simulink model "motor_dc"  (R2020b)
settings: Solver=VariableStepAuto  StartTime=0.0  StopTime=0.5  RelTol=1e-3
values from neighbouring files (symbols this model uses):
  b = 1.34e-6    (= 1.34e-06)    [parametres_load.m]
  J = 1.62e-6    (= 1.62e-06)    [parametres_load.m]
  kb = 0.011    [parametres_load.m]
  kt = 0.011    [parametres_load.m]
  La = 0.58e-3    (= 0.00058)    [parametres_load.m]
  Ra = 1.17    [parametres_load.m]
settings Model: Creator=leo7s  LastModifiedBy=leo7s

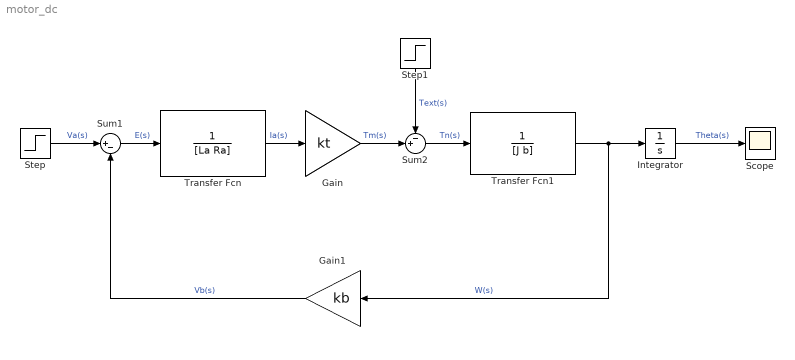
== system motor_dc ==
  Gain : Gain  Gain=kt
  Gain1 : Gain  Gain=kb
  Integrator : Integrator
  Scope : Scope
  Step : Step  Time=0  After=12  SampleTime=0
  Step1 : Step  Time=0  After=0  SampleTime=0
  Sum1 : Sum  Inputs=|+-
  Sum2 : Sum  Inputs=-+|
  Transfer Fcn : TransferFcn  Denominator=[La Ra]
  Transfer Fcn1 : TransferFcn  Denominator=[J b]
  wires:
  Step/1 -> Sum1/1  "Va(s)"
  Sum1/1 -> Transfer Fcn/1  "E(s)"
  Transfer Fcn/1 -> Gain/1  "Ia(s)"
  Gain/1 -> Sum2/2  "Tm(s)"
  Step1/1 -> Sum2/1  "Text(s)"
  Sum2/1 -> Transfer Fcn1/1  "Tn(s)"
  Gain1/1 -> Sum1/2  "Vb(s)"
  Transfer Fcn1/1 -> Gain1/1, Integrator/1  "W(s)"
  Integrator/1 -> Scope/1  "Theta(s)"
